simulink model "Proposed_method Simulink model"  (R2017a)
settings: Solver=ode45  StartTime=0.0  StopTime=10  RelTol=1e-6
undefined symbols (not defined in the file): param
settings Model: Creator=patilomkarsudhir  LastModifiedBy=Win10
settings SolverCC: ZeroCrossAlgorithm=Adaptive
settings SFSimCC: SimUseLocalCustomCode=on
settings RTWCC: RTWUseLocalCustomCode=on

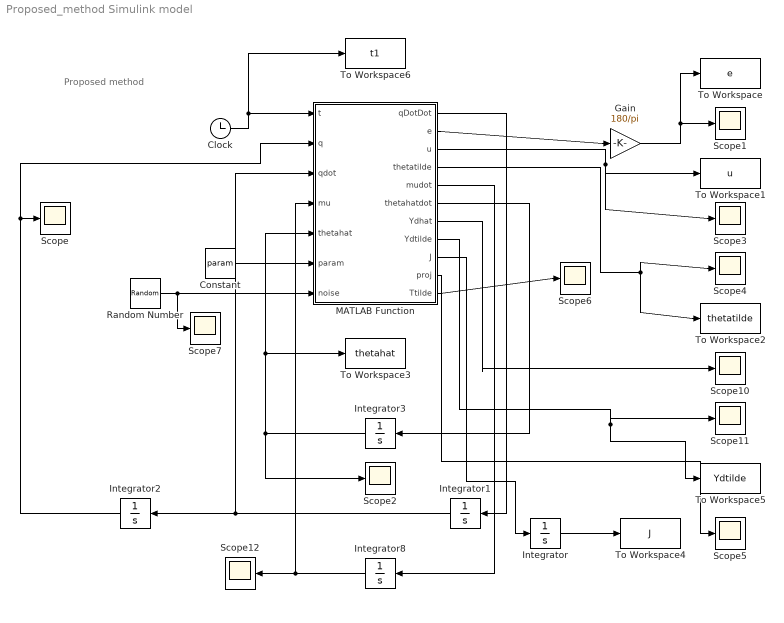
== system Proposed_method Simulink model ==
  note: Proposed method
  Clock : Clock
  Constant : Constant  Value=param
  Gain : Gain  Gain=180/pi
  Integrator : Integrator
  Integrator1 : Integrator  InitialCondition=[0;0]
  Integrator2 : Integrator  InitialCondition=[-1;1]
  Integrator3 : Integrator  InitialCondition=zeros(7,1)
  Integrator8 : Integrator  InitialCondition=[0;0]
  MATLAB Function : MATLAB Function  TreatAsAtomicUnit=on
  Random Number : RandomNumber  Mean=[0;0;0;0]  Variance=(deg2rad(2)^2)*[1;1;1;1]  SampleTime=0.01  VectorParams1D=off
  Scope{,1..7,10..12} (11 alike) : Scope
  To Workspace : ToWorkspace  VariableName=e  SampleTime=-1
  To Workspace1 : ToWorkspace  VariableName=u  SampleTime=-1
  To Workspace2 : ToWorkspace  VariableName=thetatilde  SampleTime=-1
  To Workspace3 : ToWorkspace  VariableName=thetahat  SampleTime=-1
  To Workspace4 : ToWorkspace  VariableName=J  SampleTime=-1
  To Workspace5 : ToWorkspace  VariableName=Ydtilde  SampleTime=-1
  To Workspace6 : ToWorkspace  VariableName=t1  SampleTime=-1
  wires:
  MATLAB Function/7(Ydhat) -> Scope10/1
  Integrator1/1 -> Integrator2/1, MATLAB Function/3(qdot)
  MATLAB Function/4(thetatilde) -> To Workspace2/1, Scope4/1
  MATLAB Function/8(Ydtilde) -> To Workspace5/1, Scope11/1
  MATLAB Function/2(e) -> Gain/1
  Gain/1 -> Scope1/1, To Workspace/1
  MATLAB Function/1(qDotDot) -> Integrator1/1
  Integrator8/1 -> Scope12/1, MATLAB Function/4(mu)
  Integrator3/1 -> Scope2/1, To Workspace3/1, MATLAB Function/5(thetahat)
  MATLAB Function/5(mudot) -> Integrator8/1
  Clock/1 -> To Workspace6/1, MATLAB Function/1(t)
  MATLAB Function/3(u) -> Scope3/1, To Workspace1/1
  MATLAB Function/6(thetahatdot) -> Integrator3/1
  Constant/1 -> MATLAB Function/6(param)
  MATLAB Function/9(J) -> Integrator/1
  Integrator/1 -> To Workspace4/1
  MATLAB Function/10(proj) -> Scope5/1
  MATLAB Function/11(Ttilde) -> Scope6/1
  Integrator2/1 -> MATLAB Function/2(q), Scope/1
  Random Number/1 -> Scope7/1, MATLAB Function/7(noise)

== matlab function Proposed_method Simulink model/MATLAB Function ==
  data: t input; q input; qdot input; qDotDot output; e output; u output; thetatilde output; mu input; mudot output; thetahatdot output; thetahat input; Ydhat output; Ydtilde output; param input; J output; proj output; Ttilde output; noise input
function [qDotDot,e,u,thetatilde,mudot,thetahatdot,Ydhat,Ydtilde,J,proj,Ttilde]  = fcn(t,q,qdot,mu,thetahat,param,noise)
qd=[cos(0.5*t);2*cos(t)];
qdDot=[-0.5*sin(0.5*t);-2*sin(t)];
qdDotDot=[-0.25*cos(0.5*t);-2*cos(t)];
qdDotDotDot=[0.125*sin(0.5*t);2*sin(t)];
qdDotDotDotDot=[0.0625*cos(0.5*t);2*cos(t)];
qd0=[1;2];
qdDot0=[0;0];

% Adding AWG noise to the q vector. Uncomment below 2 lines to check for AWG performance. 
% q=q+noise(1:2);
% qdot=qdot+noise(3:4);

q1=q(1);
q2=q(2);
q1dot=qdot(1);
q2dot=qdot(2);
c2=cos(q2);
s2=sin(q2);
q10=-1;
q20=1;
q1dot0=0;
q2dot0=0;
c20=cos(q20);
s20=sin(q20);
c2d=cos(qd(2));
s2d=sin(qd(2));
c2d0=cos(qd0(2));
s2d0=sin(qd0(2));
e=q-qd;
q0=[q10;q20];
qdot0=[q1dot0;q2dot0];
e10=q0-qd0;
e1dot0=qdot0-qdDot0;
edot=qdot-qdDot;
e1=e;
e1dot=edot;
% alpha=1;
k=param(1);
beta=param(2);
alpha=param(3);
alpha2=param(4);
e2=e1dot+alpha*e1;
e20=e1dot0+alpha*e10;



Yd=[qdDotDot(1) qdDotDot(2) 2*c2d*qdDotDot(1)+c2d*qdDotDot(2)-s2d*qdDot(1)*qdDot(2)-s2d*(qdDot(1)+qdDot(2))*qdDot(2) qdDot(1) 0;
    0 qdDotDot(1)+qdDotDot(2) s2d*qdDot(1)^2+c2d*qdDotDot(2) 0 qdDot(2)];
Yd=[Yd eye(length(e))];

Gamma=1;
% k=0.01;
% alpha2=0.1;


thetabar=5000;
f=norm(thetahat)^2-thetabar^2;
delf=2*thetahat;
prjscl=delf*delf'/norm(delf)^2;
Lambda=Yd'*inv(Yd*Yd')*(k*alpha2*e2+beta*sign(e2));
if((f<0)||(delf'*Lambda<=0))
    thetahatdot=Lambda;
    mudot=[0;0];
    proj=0;
else
    thetahatdot=(eye(length(thetahat))-prjscl)*Lambda;
    mudot=-Yd*prjscl*Lambda;
    proj=1;
end
mu=mu-k*e2;



u=-Yd*thetahat+mu;


p1 = 3.473+0.5*sin(3*t);
p2 = 0.196+0.2*exp(-sin(t));
p3 = 0.242+0.1*cos(10*t);

fd1 = 5.3+2*exp(-0.1*t);
fd2 = 1.1+cos(5*t);
theta=[p1;p2;p3;fd1;fd2];
disturbance=[0.5*cos(0.5*t);sin(t)];
theta=[theta;disturbance];
thetatilde=theta+thetahat;
M = [p1+2*p3*cos(q(2)), p2+p3*cos(q(2)); p2+p3*cos(q(2)), p2];
Vm = [-p3*sin(q(2))*qdot(2), -p3*sin(q(2))*(qdot(1)+qdot(2)); p3*sin(q(2))*qdot(1), 0];
Fd = [fd1, 0; 0, fd2];

qDotDot = M\(u - Vm*qdot - Fd*qdot-disturbance);
Ydhat=Yd*thetahat;
Ydtilde=u+Yd*thetahat;
J=0.01*norm(u)^2+norm(e)^2;
qDot=qdot;
Y=[qDotDot(1) qDotDot(2) 2*c2*qDotDot(1)+c2*qDotDot(2)-s2*qDot(1)*qDot(2)-s2*(qDot(1)+qDot(2))*qDot(2) qDot(1) 0 1 0;
    0 qDotDot(1)+qDotDot(2) s2*qDot(1)^2+c2*qDotDot(2) 0 qDot(2) 0 1];
Ttilde=u-Y*theta;
